simulink library "INT_FlCDspl_DD"  (R2016b)
settings: Solver=VariableStepAuto  StartTime=0.0  StopTime=10.0  RelTol=1e-3
settings Model: Creator=Wei Liang  LastModifiedBy=Wei Liang

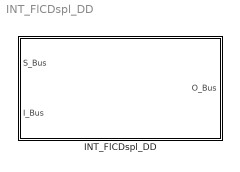
== system INT_FlCDspl_DD ==
  INT_FlCDspl_DD : Subsystem

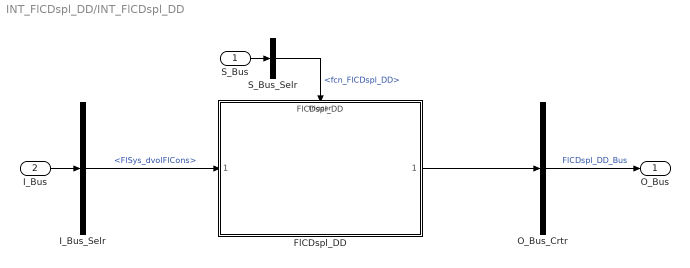
== system INT_FlCDspl_DD/INT_FlCDspl_DD ==
  S_Bus : Inport
  I_Bus : Inport  Port=2
  FlCDspl_DD : ModelReference  ModelNameDialog=FlCDspl_DD  SimulationMode=Normal  ModelReferenceVersion=1.16  TriggerPortName=function  TriggerPortTriggerType=function-call  TriggerPortStatesWhenEnabling=held
  I_Bus_Selr : BusSelector  OutputSignals=FlSys_dvolFlCons
  O_Bus_Crtr : BusCreator  Inputs=1
  S_Bus_Selr : BusSelector  OutputSignals=fcn_FlCDspl_DD
  O_Bus : Outport
  wires:
  S_Bus_Selr/1 -> FlCDspl_DD/Trigger  "<fcn_FlCDspl_DD>"
  S_Bus/1 -> S_Bus_Selr/1
  I_Bus/1 -> I_Bus_Selr/1
  I_Bus_Selr/1 -> FlCDspl_DD/1  "<FlSys_dvolFlCons>"
  O_Bus_Crtr/1 -> O_Bus/1  "FlCDspl_DD_Bus"
  FlCDspl_DD/1 -> O_Bus_Crtr/1
